simulink model "CounterUpWithResetButton"  (R2024b)
settings: Solver=VariableStepAuto  StartTime=0.0  StopTime=10.0  RelTol=1e-3
settings Model: Creator=MOHAMED  LastModifiedBy=MOHAMED

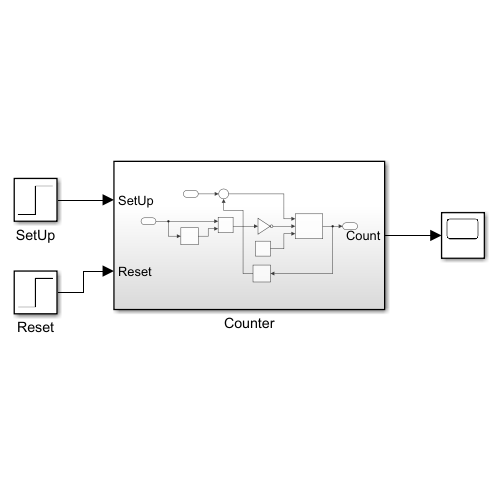
[thumbnail: Simulink's stored preview of the top-level diagram]
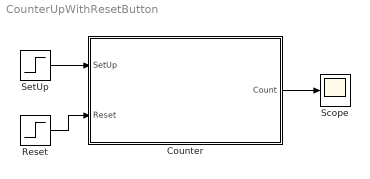
== system CounterUpWithResetButton ==
  Counter : Subsystem
  Reset : Step  Time=5  SampleTime=0
  Scope : Scope
  SetUp : Step  SampleTime=0
  wires:
  SetUp/1 -> Counter/1(SetUp)
  Reset/1 -> Counter/2(Reset)
  Counter/1(Count) -> Scope/1

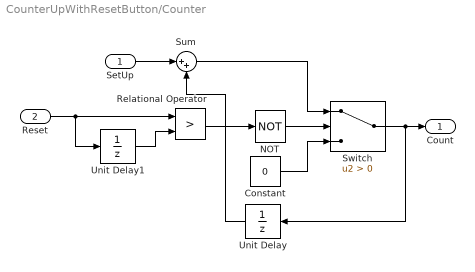
== system CounterUpWithResetButton/Counter ==
  SetUp : Inport
  Reset : Inport  Port=2
  Constant : Constant  Value=0
  NOT : Logic  Operator=NOT  IconShape=distinctive  AllPortsSameDT=off  OutDataTypeStr=boolean
  Relational Operator : RelationalOperator  Operator=>  OutDataTypeStr=boolean  RndMeth=Simplest  InputSameDT=off
  Sum : Sum  Inputs=|++
  Switch : Switch  Criteria=u2 > Threshold  SaturateOnIntegerOverflow=off  InputSameDT=off
  Unit Delay : UnitDelay  SampleTime=-1  HasFrameUpgradeWarning=on
  Unit Delay1 : UnitDelay  SampleTime=-1  HasFrameUpgradeWarning=on
  Count : Outport
  wires:
  Unit Delay/1 -> Sum/2
  Reset/1 -> Relational Operator/1, Unit Delay1/1
  SetUp/1 -> Sum/1
  Relational Operator/1 -> NOT/1
  Unit Delay1/1 -> Relational Operator/2
  Constant/1 -> Switch/3
  NOT/1 -> Switch/2
  Sum/1 -> Switch/1
  Switch/1 -> Unit Delay/1, Count/1
